simulink model "Tmod_PID_ObsMej_Simulacion"  (R2021a)
settings: Solver=VariableStepAuto  StartTime=0.0  StopTime=20  MaxStep=1e-4  RelTol=1e-3
values from neighbouring files (symbols this model uses):
  a1c = -A1(2, 2)    [filtros_ss.m]
  a1m = -A4(2, 2)    [filtros_ss.m]
  a1p = -A2(2, 2)    [filtros_ss.m]
  a1t = -A3    [filtros_ss.m]
  a2c = -A1(2, 1)    [filtros_ss.m]
  a2m = -A4(2, 1)    [filtros_ss.m]
  a2p = -A2(2, 1)    [filtros_ss.m]
  a_cu = 3.9e-3    (= 0.0039)    [Datos.m]
  b_eq = 15.000e-6    (= 1.5e-05)    [Datos.m]
  ba = 0.0113    [Datos.m]
  Cts = 0.818    [Datos.m]
  Id_0 = 0    [Datos.m]
  J_eq = 5.6509e-6    (= 5.6509e-06)    [Datos.m]
  Ksa = 9.0414    [Datos.m]
  Ksia = 2893.2608    [Datos.m]
  lambda_m = 0.01546    [Datos.m]
  Ld = 6.6e-3    (= 0.0066)    [Datos.m]
  Lls = 0.8e-3    (= 0.0008)    [Datos.m]
  Lq = 5.8e-3    (= 0.0058)    [Datos.m]
  Pp = 3.01    [Datos.m]
  r = 314.3008    [Datos.m]
  Rs = 1.02    [Datos.m]
  Rs_ref = 1.02    [Datos.m]
  Rtsamb = 146.7    [Datos.m]
  sat = sqrt(2/3)*24    [filtros_ss.m]
  T_0 = 40.0    (= 40)    [Datos.m]
  T_amb = 40    [Datos.m]
  Tlmax = 6.28    [Datos.m]
  Ts_ref = 40    [Datos.m]
undefined symbols (not defined in the file or in its folder): A1, A2, A3, B1, B2, B3, C1, C2, C3, D1, D2, D3, mKi, mKtheta, mKw, R0, Rd, Rq, sigbuilder_block
libraries: simulink x1
settings Model: Creator=ThnkPad  LastModifiedBy=jpss8

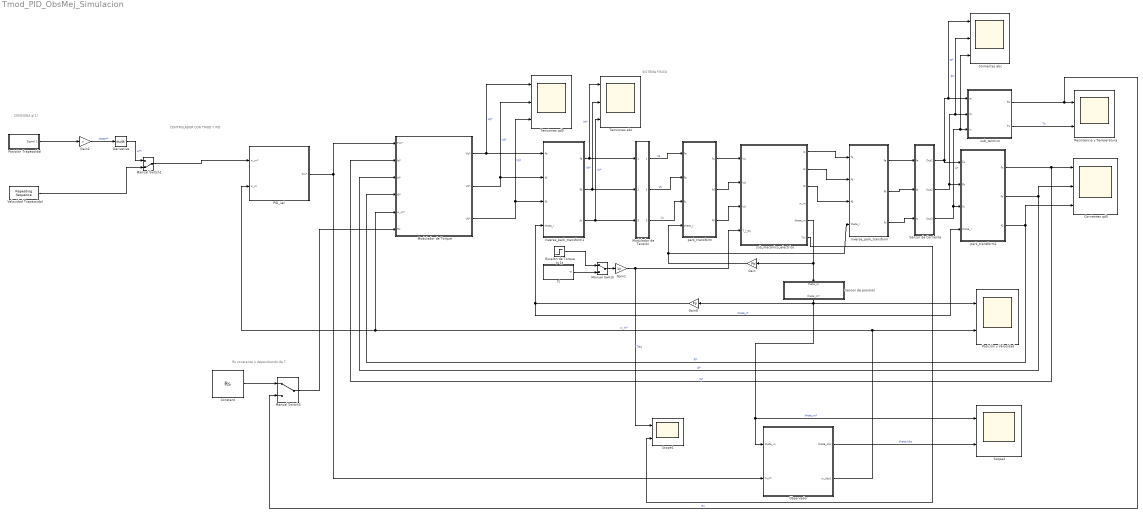
== system Tmod_PID_ObsMej_Simulacion ==
  note: Rs constante o dependiendo de T
  note: CONSIGNA q(1)
  note: CONTROLADOR CON TMOD Y PID
  note: SISTEMA FÍSICO
  Constant : Constant  Value=Rs
  Corrientes abc : Scope  NumInputPorts=3
  Corrientes qd0 : Scope  NumInputPorts=3
  Derivative : Derivative
  Escalón de Torque t=1s : Step  After=Tlmax  SampleTime=0
  Gain : Gain  Gain=Pp
  Gain1 : Gain  Gain=1/r
  Gain2 : Gain  Gain=r
  Gain8 : Gain  Gain=Pp
  Manual Switch : ManualSwitch
  Manual Switch1 : ManualSwitch  CurrentSetting=0
  Manual Switch3 : ManualSwitch
  Modulador de Tensión : Subsystem
  Modulador de Torque : Subsystem
  Observador : Subsystem
  PID_vel : Subsystem
  Posición Trapezoidal : Subsystem  Tag=STV Subsys  LoadFcn=sigbuilder_block('load');  StartFcn=sigbuilder_block('start');  StopFcn=sigbuilder_block('stop');  ClipboardFcn=sigbuilder_block('clipboard');  mask(Sigbuilder block){tuvar=[0:10]}
      mask help: Simulink:masks:SigbuilderBlock_MD
      mask init:
      | if ~strcmp(get_param(bdroot(gcbh),'SimulationStatus'),'stopped') tuvar = sigbuilder_block('maskInit'); end
      settings: CopyFcn=sigbuilder_block('copy');  DeleteFcn=sigbuilder_block('delete');  ModelCloseFcn=sigbuilder_block('modelClose');  PreSaveFcn=sigbuilder_block('preSave');  PauseFcn=sigbuilder_block('pause');  ContinueFcn=sigbuilder_block('continue');  NameChangeFcn=sigbuilder_block('namechange');  OpenFcn=sigbuilder_block('open',[-53.25 9 1012.5 477.75 ]);  CloseFcn=sigbuilder_block('close');
      mask Display: plot(0, 0, 100, 100,[2, 2, 32, 32, 2], [68, 8, 8, 68, 68],[32, 2], [38, 38], [32, 19, 2],[53, 60, 44], [32, 17, 17, 2],[16, 16, 31, 31]);txt = getActiveGroup(gcbh);text(2, 100, txt,'verticalAlignment', 'top');
  Posición y Velocidad : Scope  NumInputPorts=2
  Resistencia y Temperatura : Scope  NumInputPorts=2
  Scope1 : Scope  NumInputPorts=2
  Scope2 : Scope  NumInputPorts=2
  Sensor de Corriente : Subsystem
  Sensor de posicion : Subsystem
      settings: PortSchema="{\"entries\":[{\"content\":{\"sides\":[{\"content\":{\"connectorIds\":[]},\"type\":\"ConnectorPlacement.EquallySpacedRectSide\",\"uuid\":\"b536d0fd-a8b9-4fb9-bd2d-8cdbea63ffed\"},{\"content\":{\"connectorIds\":[],\"side\":\"RIGHT\"},\"type\":\"ConnectorPlacement.EquallySpacedRectSide\",\"uuid\":\"53663a0b-a681-499d-8c35-4379374d5e5a\"},{\"content\":{\"connectorIds\":[\"In1\"],\"side\":\"TOP\"},\"type\":\"ConnectorPlacement.EquallySpacedRectSide\",\"uuid\":\"1d4df5dd-d4dd-4e51-a644-5027fa847818\"},{\"content\":{\"connectorIds\":[\"Out1\"],\"side\":\"BOTTOM\"},\"type\":\"ConnectorPlacement.EquallySpacedRectSide\",\"uuid\":\"bae52777-b033-4852-a05b-da4dd91f0167\"}]},\"type\":\"ConnectorPlacement.EquallySpacedConnector\",\"uuid\":\"afdb905b-2ae6-4e5d-8f00-48d2cd8bae21\"}],\"packageUris\":[\"http://schema.mathworks.com/mf0/Connector/R2020b\"],\"version\":\"1.0\"}"
  Tensiones abc : Scope  NumInputPorts=3
  Tensiones qd0 : Scope  NumInputPorts=3
  Tl : Subsystem  Tag=STV Subsys  LoadFcn=sigbuilder_block('load');  StartFcn=sigbuilder_block('start');  StopFcn=sigbuilder_block('stop');  ClipboardFcn=sigbuilder_block('clipboard');  mask(Sigbuilder block){tuvar=[0:10]}
      mask help: Simulink:masks:SigbuilderBlock_MD
      mask init:
      | if ~strcmp(get_param(bdroot(gcbh),'SimulationStatus'),'stopped') tuvar = sigbuilder_block('maskInit'); end
      settings: CopyFcn=sigbuilder_block('copy');  DeleteFcn=sigbuilder_block('delete');  ModelCloseFcn=sigbuilder_block('modelClose');  PreSaveFcn=sigbuilder_block('preSave');  PauseFcn=sigbuilder_block('pause');  ContinueFcn=sigbuilder_block('continue');  NameChangeFcn=sigbuilder_block('namechange');  OpenFcn=sigbuilder_block('open',[6 0 1012.5 477.75 ]);  CloseFcn=sigbuilder_block('close');
      mask Display: plot(0, 0, 100, 100,[2, 2, 32, 32, 2], [68, 8, 8, 68, 68],[32, 2], [38, 38], [32, 19, 2],[53, 60, 44], [32, 17, 17, 2],[16, 16, 31, 31]);txt = getActiveGroup(gcbh);text(2, 100, txt,'verticalAlignment', 'top');
  Velocidad Trapezoidal : simulink/Sources/Repeating Sequence  rep_seq_t=t_sequence  rep_seq_y=w2
  inverse_park_transform : MATLAB Function  TreatAsAtomicUnit=on
  inverse_park_transform1 : MATLAB Function  TreatAsAtomicUnit=on
  park_transform : MATLAB Function  TreatAsAtomicUnit=on
  park_transform1 : MATLAB Function  TreatAsAtomicUnit=on
  sub_mecanico_electrico : Subsystem
  sub_termico : Subsystem
  wires:
  Sensor de Corriente/3(Out3) -> park_transform1/3(fc), Corrientes abc/3, sub_termico/3(ic)  "Ic*"
  sub_termico/2(Ts) -> Resistencia y Temperatura/2  "Ts"
  inverse_park_transform1/2(fb) -> Modulador de Tensión/2(Vb), Tensiones abc/2  "Vb*"
  Modulador de Torque/2(Vd*) -> Tensiones qd0/2, inverse_park_transform1/2(fd)  "Vd*"
  Sensor de Corriente/2(Out2) -> park_transform1/2(fb), Corrientes abc/2, sub_termico/2(ib)  "Ib*"
  PID_vel/1(Tm*) -> Modulador de Torque/1(Tm*'), Observador/2(Tm**)
  park_transform1/3(f0) -> Corrientes qd0/3, Modulador de Torque/4(I0*)  "I0*"
  park_transform1/1(fq) -> Modulador de Torque/2(Iq*), Corrientes qd0/1  "Iq*"
  inverse_park_transform1/1(fa) -> Tensiones abc/1, Modulador de Tensión/1(Va)  "Va*"
  Modulador de Torque/3(V0*) -> inverse_park_transform1/3(f0), Tensiones qd0/3  "V0*"
  Gain/1 -> inverse_park_transform/4(theta_r), park_transform/4(theta_r)
  sub_mecanico_electrico/5(theta_m) -> Sensor de posicion/1(theta_m), Gain/1
  inverse_park_transform1/3(fc) -> Modulador de Tensión/3(Vc), Tensiones abc/3  "Vc*"
  inverse_park_transform/1(fa) -> Sensor de Corriente/1(Ia)
  inverse_park_transform/3(fc) -> Sensor de Corriente/3(Ic)
  park_transform/2(fd) -> sub_mecanico_electrico/2(Vd)
  sub_mecanico_electrico/1(iq) -> inverse_park_transform/1(fq)
  park_transform1/2(fd) -> Corrientes qd0/2, Modulador de Torque/3(Id*)  "Id*"
  Gain8/1 -> park_transform1/4(theta_r), inverse_park_transform1/4(theta_r)  "theta_r*"
  park_transform/1(fq) -> sub_mecanico_electrico/1(Vq)
  park_transform/3(f0) -> sub_mecanico_electrico/3(V0)
  Sensor de posicion/1(theta_m*) -> Posición y Velocidad/1, Scope2/1, Observador/1(theta_m), Gain8/1  "theta_m*"
  Modulador de Torque/1(Vq*) -> Tensiones qd0/1, inverse_park_transform1/1(fq)  "Vq*"
  Modulador de Tensión/3(Vc*) -> park_transform/3(fc)  "Vc"
  Sensor de Corriente/1(Out1) -> park_transform1/1(fa), Corrientes abc/1, sub_termico/1(ia)  "Ia*"
  inverse_park_transform/2(fb) -> Sensor de Corriente/2(Ib)
  sub_termico/1(Rs) -> Resistencia y Temperatura/1, Manual Switch3/2  "Rs"
  Modulador de Tensión/1(Va*) -> park_transform/1(fa)  "Va"
  Observador/2(w_obs1) -> PID_vel/2(w_m), Modulador de Torque/5(w_m*), Posición y Velocidad/2  "w_m*"
  Modulador de Tensión/2(Vb*) -> park_transform/2(fb)  "Vb"
  sub_mecanico_electrico/3(i0) -> inverse_park_transform/3(f0)
  Gain1/1 -> Scope1/1, sub_mecanico_electrico/4(T_l_eq)  "Tleq"
  sub_mecanico_electrico/2(id) -> inverse_park_transform/2(fd)
  Gain2/1 -> Derivative/1  "theta**"
  sub_mecanico_electrico/6(Tm) -> Scope1/2
  Observador/1(theta_obs) -> Scope2/2  "theta_obs"
  Tl/1(Tl) -> Manual Switch/2
  Escalón de Torque t=1s/1 -> Manual Switch/1
  Posición Trapezoidal/1(Signal 1) -> Gain2/1
  Constant/1 -> Manual Switch3/1
  Manual Switch3/1 -> Modulador de Torque/6(Rs)
  Manual Switch1/1 -> PID_vel/1(w_m*)
  Derivative/1 -> Manual Switch1/1  "w**"
  Velocidad Trapezoidal/1 -> Manual Switch1/2
  Manual Switch/1 -> Gain1/1

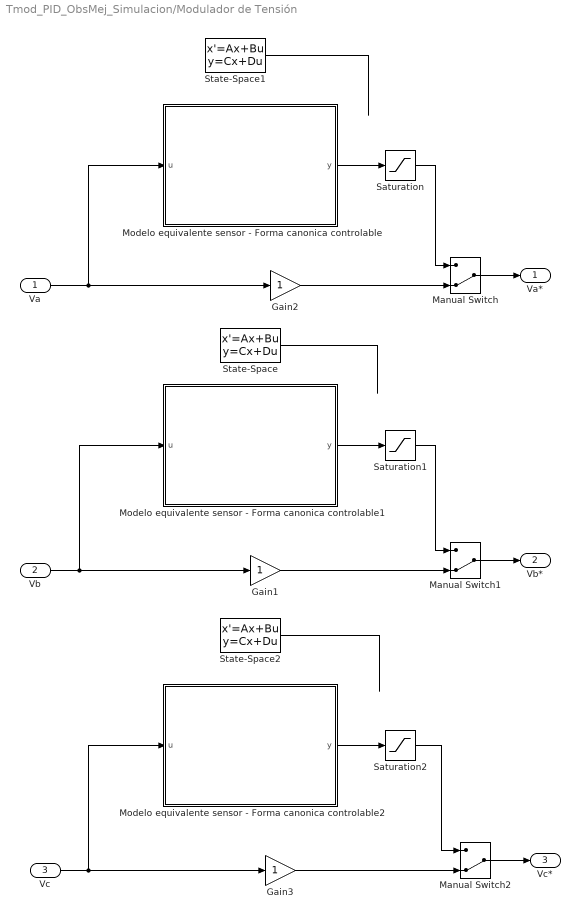
== system Tmod_PID_ObsMej_Simulacion/Modulador de Tensión ==
  Va : Inport
  Vb : Inport  Port=2
  Vc : Inport  Port=3
  Gain1 : Gain
  Gain2 : Gain
  Gain3 : Gain
  Manual Switch : ManualSwitch  CurrentSetting=0
  Manual Switch1 : ManualSwitch  CurrentSetting=0
  Manual Switch2 : ManualSwitch  CurrentSetting=0
  Modelo equivalente sensor - Forma canonica controlable : Subsystem
  Modelo equivalente sensor - Forma canonica controlable1 : Subsystem
  Modelo equivalente sensor - Forma canonica controlable2 : Subsystem
  Saturation : Saturate  UpperLimit=sat  LowerLimit=-sat
  Saturation1 : Saturate  UpperLimit=sat  LowerLimit=-sat
  Saturation2 : Saturate  UpperLimit=sat  LowerLimit=-sat
  State-Space : StateSpace  A=A1  B=B1  C=C1  D=D1  InitialCondition=0
  State-Space1 : StateSpace  A=A1  B=B1  C=C1  D=D1  InitialCondition=0
  State-Space2 : StateSpace  A=A1  B=B1  C=C1  D=D1  InitialCondition=0
  Va* : Outport
  Vb* : Outport  Port=2
  Vc* : Outport  Port=3
  wires:
  Va/1 -> Modelo equivalente sensor - Forma canonica controlable/1(u), Gain2/1
  Manual Switch/1 -> Va*/1
  Gain2/1 -> Manual Switch/2
  Vb/1 -> Modelo equivalente sensor - Forma canonica controlable1/1(u), Gain1/1
  Manual Switch1/1 -> Vb*/1
  Gain1/1 -> Manual Switch1/2
  Vc/1 -> Modelo equivalente sensor - Forma canonica controlable2/1(u), Gain3/1
  Manual Switch2/1 -> Vc*/1
  Gain3/1 -> Manual Switch2/2
  Saturation/1 -> Manual Switch/1
  Saturation1/1 -> Manual Switch1/1
  Saturation2/1 -> Manual Switch2/1
  State-Space/1 -> ?
  State-Space1/1 -> ?
  State-Space2/1 -> ?
  Modelo equivalente sensor - Forma canonica controlable/1(y) -> Saturation/1
  Modelo equivalente sensor - Forma canonica controlable1/1(y) -> Saturation1/1
  Modelo equivalente sensor - Forma canonica controlable2/1(y) -> Saturation2/1

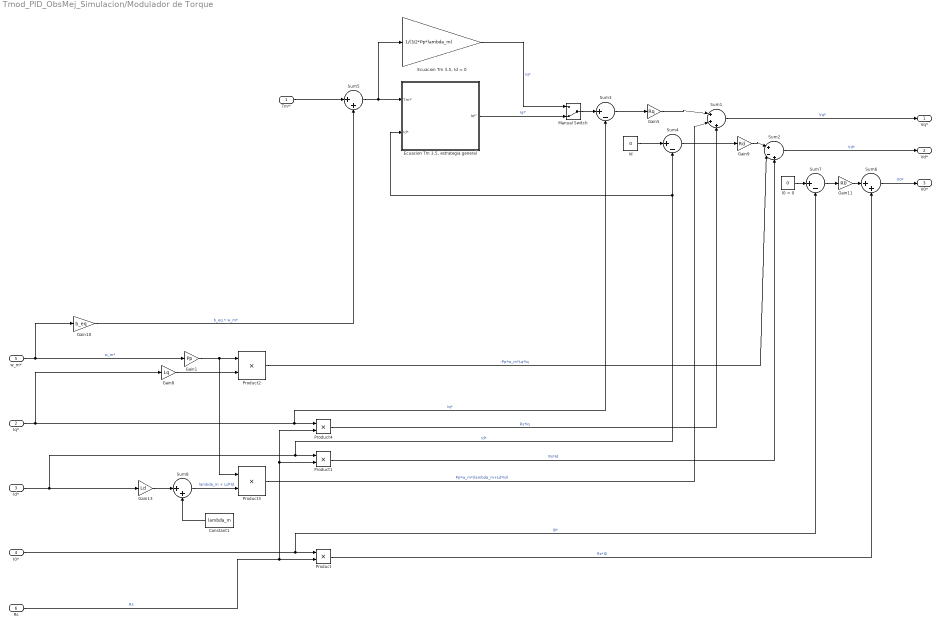
== system Tmod_PID_ObsMej_Simulacion/Modulador de Torque ==
  Tm*' : Inport
  Iq* : Inport  Port=2
  Id* : Inport  Port=3
  I0* : Inport  Port=4
  w_m* : Inport  Port=5
  Rs : Inport  Port=6
  Constant1 : Constant  Value=lambda_m
  "Ecuacion Tm 3.5, Id = 0" : Gain  Gain=1/(3/2*Pp*lambda_m)
  "Ecuacion Tm 3.5, estrategia general" : Subsystem
  Gain1 : Gain  Gain=Pp
  Gain10 : Gain  Gain=b_eq
  Gain11 : Gain  Gain=R0
  Gain13 : Gain  Gain=Ld
  Gain5 : Gain  Gain=Rq
  Gain8 : Gain  Gain=Lq
  Gain9 : Gain  Gain=Rd
  I0 = 0 : Constant  Value=0
  Id : Constant  Value=0
  Manual Switch : ManualSwitch  CurrentSetting=0
  Product{,1..4} (5 alike) : Product
  Sum1 : Sum  Inputs=|+++
  Sum2 : Sum  Inputs=|+-+
  Sum3 : Sum  Inputs=|+-
  Sum4 : Sum  Inputs=|+-
  Sum5 : Sum  Inputs=|++
  Sum6 : Sum  Inputs=|++
  Sum7 : Sum  Inputs=|+-
  Sum8 : Sum  Inputs=|++
  Vq* : Outport
  Vd* : Outport  Port=2
  V0* : Outport  Port=3
  wires:
  Sum7/1 -> Gain11/1
  I0 = 0/1 -> Sum7/1
  Tm*'/1 -> Sum5/1
  "Ecuacion Tm 3.5, Id = 0"/1 -> Manual Switch/1  "Iq*"
  Sum4/1 -> Gain9/1
  Sum5/1 -> "Ecuacion Tm 3.5, Id = 0"/1, "Ecuacion Tm 3.5, estrategia general"/1(Tm*')
  Id/1 -> Sum4/1
  Gain5/1 -> Sum1/1
  Gain9/1 -> Sum2/1
  Sum3/1 -> Gain5/1
  Sum2/1 -> Vd*/1  "Vd*"
  Gain11/1 -> Sum6/1
  Sum1/1 -> Vq*/1  "Vq*"
  Gain10/1 -> Sum5/2  "b_eq * w_m*"
  Product4/1 -> Sum1/3  "Rs*Iq"
  Product2/1 -> Sum2/2  "-Pp*w_m*Lq*Iq"
  Product1/1 -> Sum2/3  "Rs*Id"
  Product/1 -> Sum6/2  "Rs*I0"
  Product3/1 -> Sum1/2  "Pp*w_m*(lambda_m+Ld*Id)"
  w_m*/1 -> Gain10/1, Gain1/1  "w_m*"
  Iq*/1 -> Product4/1, Sum3/2, Gain8/1  "Iq*"
  Gain13/1 -> Sum8/1
  Gain8/1 -> Product2/2
  Gain1/1 -> Product3/1, Product2/1
  Constant1/1 -> Sum8/2
  Sum8/1 -> Product3/2  "lambda_m + Ld*Id"
  Id*/1 -> Product1/1, "Ecuacion Tm 3.5, estrategia general"/2(Id*), Sum4/2, Gain13/1  "Id*"
  I0*/1 -> Product/1, Sum7/2  "I0*"
  Sum6/1 -> V0*/1  "V0*"
  "Ecuacion Tm 3.5, estrategia general"/1(Iq*') -> Manual Switch/2  "Iq*'"
  Manual Switch/1 -> Sum3/1
  Rs/1 -> Product1/2, Product4/2, Product/2  "Rs"

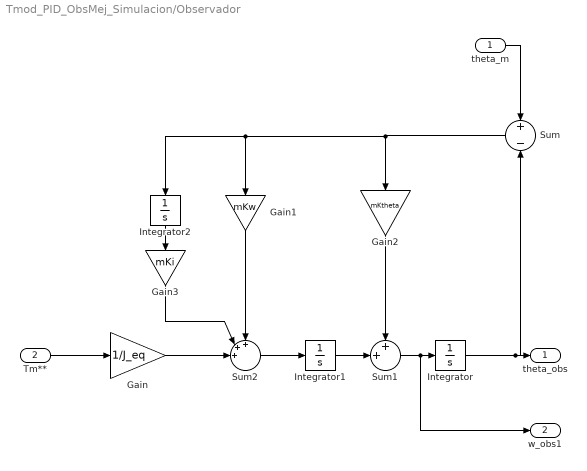
== system Tmod_PID_ObsMej_Simulacion/Observador ==
  theta_m : Inport
  Tm** : Inport  Port=2
  Gain : Gain  Gain=1/J_eq
  Gain1 : Gain  Gain=mKw
  Gain2 : Gain  Gain=mKtheta
  Gain3 : Gain  Gain=mKi
  Integrator : Integrator
  Integrator1 : Integrator
  Integrator2 : Integrator
  Sum : Sum  Inputs=+|-
  Sum1 : Sum  Inputs=++|
  Sum2 : Sum  Inputs=+++||
  theta_obs : Outport
  w_obs1 : Outport  Port=2
  wires:
  Integrator/1 -> Sum/2, theta_obs/1
  Sum2/1 -> Integrator1/1
  Sum/1 -> Integrator2/1, Gain1/1, Gain2/1
  theta_m/1 -> Sum/1
  Tm**/1 -> Gain/1
  Gain1/1 -> Sum2/1
  Gain2/1 -> Sum1/1
  Integrator1/1 -> Sum1/2
  Sum1/1 -> w_obs1/1, Integrator/1
  Gain/1 -> Sum2/3
  Gain3/1 -> Sum2/2
  Integrator2/1 -> Gain3/1

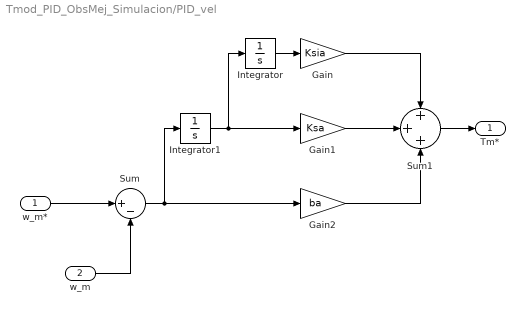
== system Tmod_PID_ObsMej_Simulacion/PID_vel ==
  w_m* : Inport
  w_m : Inport  Port=2
  Gain : Gain  Gain=Ksia
  Gain1 : Gain  Gain=Ksa
  Gain2 : Gain  Gain=ba
  Integrator : Integrator
  Integrator1 : Integrator
  Sum : Sum  Inputs=|+-
  Sum1 : Sum  Inputs=+++
  Tm* : Outport
  wires:
  Gain1/1 -> Sum1/2
  Sum1/1 -> Tm*/1
  Sum/1 -> Integrator1/1, Gain2/1
  Integrator/1 -> Gain/1
  Gain2/1 -> Sum1/3
  Gain/1 -> Sum1/1
  Integrator1/1 -> Gain1/1, Integrator/1
  w_m*/1 -> Sum/1
  w_m/1 -> Sum/2

== system Tmod_PID_ObsMej_Simulacion/Posición Trapezoidal ==
  Demux : Demux  Tag=STV Demux  Outputs=1
      settings: DisplayOption=none
  FromWs : FromWorkspace  Tag=STV FromWs  VariableName=tuvar
      SigBuilderData=|
      | common.afterFinalStr = 'Extrapolate'
      | common.sampleTime = 0
      | dataSet.timeRange = [0 20]
      | dataSet.name = 'Group 1'
      | sbobj.Groups.Name = 'Group 1'
      | sbobj.Groups.Signals.Name = 'Signal 1'
      | sbobj.Groups.Signals.XData = [0 2 7 12 17 20]
      | sbobj.Groups.Signals.YData = [0 0 6.28318530718 6.28318530718 0 0]
      | sbobj.Groups.TimeRange = [0 20]
  Signal 1 : Outport  Tag=STV Outport
  wires:
  Demux/1 -> Signal 1/1
  FromWs/1 -> Demux/1

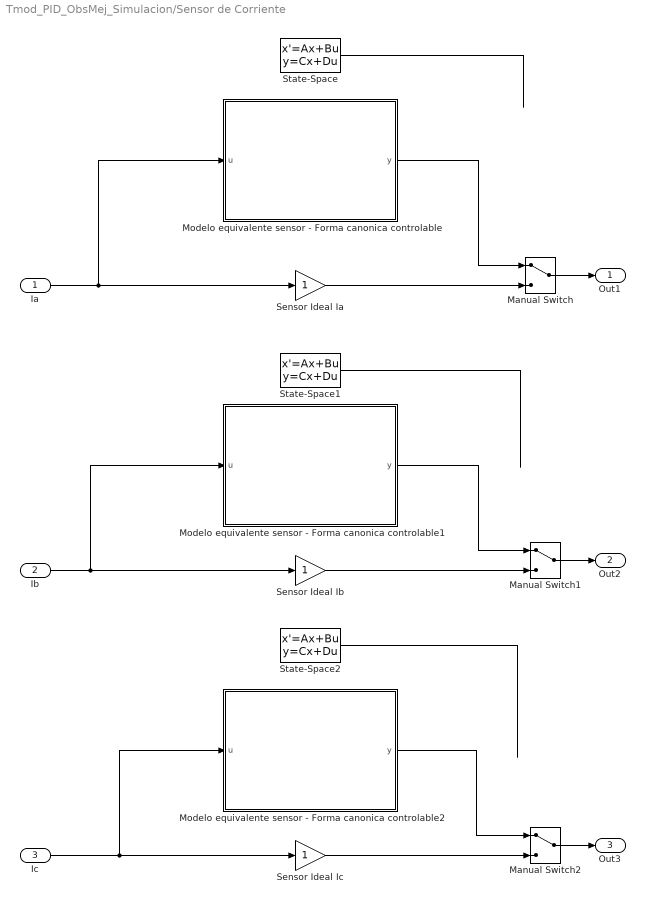
== system Tmod_PID_ObsMej_Simulacion/Sensor de Corriente ==
  Ia : Inport
  Ib : Inport  Port=2
  Ic : Inport  Port=3
  Manual Switch : ManualSwitch
  Manual Switch1 : ManualSwitch
  Manual Switch2 : ManualSwitch
  Modelo equivalente sensor - Forma canonica controlable : Subsystem
  Modelo equivalente sensor - Forma canonica controlable1 : Subsystem
  Modelo equivalente sensor - Forma canonica controlable2 : Subsystem
  Sensor Ideal Ia : Gain
  Sensor Ideal Ib : Gain
  Sensor Ideal Ic : Gain
  State-Space : StateSpace  A=A1  B=B1  C=C1  D=D1  InitialCondition=0
  State-Space1 : StateSpace  A=A1  B=B1  C=C1  D=D1  InitialCondition=0
  State-Space2 : StateSpace  A=A1  B=B1  C=C1  D=D1  InitialCondition=0
  Out1 : Outport
  Out2 : Outport  Port=2
  Out3 : Outport  Port=3
  wires:
  Ic/1 -> Modelo equivalente sensor - Forma canonica controlable2/1(u), Sensor Ideal Ic/1
  Ib/1 -> Modelo equivalente sensor - Forma canonica controlable1/1(u), Sensor Ideal Ib/1
  Ia/1 -> Modelo equivalente sensor - Forma canonica controlable/1(u), Sensor Ideal Ia/1
  Manual Switch/1 -> Out1/1
  Sensor Ideal Ia/1 -> Manual Switch/2
  Manual Switch2/1 -> Out3/1
  Manual Switch1/1 -> Out2/1
  Sensor Ideal Ib/1 -> Manual Switch1/2
  Sensor Ideal Ic/1 -> Manual Switch2/2
  State-Space/1 -> ?
  State-Space1/1 -> ?
  State-Space2/1 -> ?
  Modelo equivalente sensor - Forma canonica controlable/1(y) -> Manual Switch/1
  Modelo equivalente sensor - Forma canonica controlable1/1(y) -> Manual Switch1/1
  Modelo equivalente sensor - Forma canonica controlable2/1(y) -> Manual Switch2/1

== system Tmod_PID_ObsMej_Simulacion/Sensor de posicion ==
  theta_m : Inport
  Manual Switch : ManualSwitch
  Modelo equivalente sensor - Forma canonica controlable : Subsystem
  Sensor Ideal : Gain
  State-Space : StateSpace  A=A2  B=B2  C=C2  D=D2  InitialCondition=0
  theta_m* : Outport
  wires:
  theta_m/1 -> Modelo equivalente sensor - Forma canonica controlable/1(u), Sensor Ideal/1
  Manual Switch/1 -> theta_m*/1
  Sensor Ideal/1 -> Manual Switch/2
  Modelo equivalente sensor - Forma canonica controlable/1(y) -> Manual Switch/1
  State-Space/1 -> ?

== system Tmod_PID_ObsMej_Simulacion/Tl ==
  Demux : Demux  Tag=STV Demux  Outputs=1
      settings: DisplayOption=none
  FromWs : FromWorkspace  Tag=STV FromWs  VariableName=tuvar
      SigBuilderData=|
      | common.afterFinalStr = 'Extrapolate'
      | common.sampleTime = 0
      | dataSet.timeRange = [0 1]
      | dataSet.name = 'Group 1'
      | sbobj.Groups.Name = 'Group 1'
      | sbobj.Groups.Signals.Name = 'Tl'
      | sbobj.Groups.Signals.XData = [0 0.3 0.3 0.5 0.5 0.9 0.9 1]
      | sbobj.Groups.Signals.YData = [0 0 6.28 6.28 -6.28 -6.28 0 0]
      | sbobj.Groups.TimeRange = [0 1]
  Tl : Outport  Tag=STV Outport
  wires:
  FromWs/1 -> Demux/1
  Demux/1 -> Tl/1

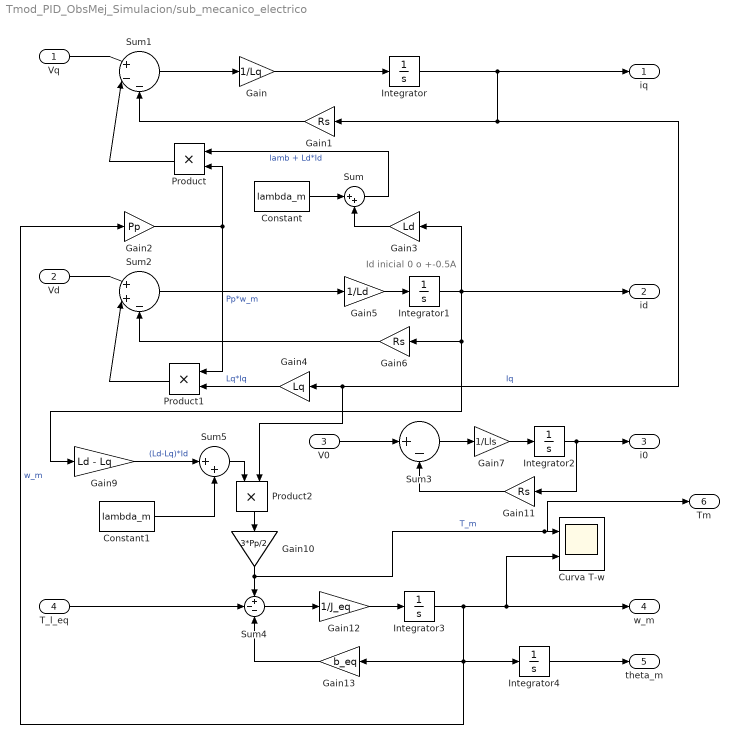
== system Tmod_PID_ObsMej_Simulacion/sub_mecanico_electrico ==
  note: Id inicial 0 o +-0.5A
  Vq : Inport
  Vd : Inport  Port=2
  V0 : Inport  Port=3
  T_l_eq : Inport  Port=4
  Constant : Constant  Value=lambda_m
  Constant1 : Constant  Value=lambda_m
  Curva T-w : Scope  NumInputPorts=2
  Gain : Gain  Gain=1/Lq
  Gain1 : Gain  Gain=Rs
  Gain10 : Gain  Gain=3*Pp/2
  Gain11 : Gain  Gain=Rs
  Gain12 : Gain  Gain=1/J_eq
  Gain13 : Gain  Gain=b_eq
  Gain2 : Gain  Gain=Pp
  Gain3 : Gain  Gain=Ld
  Gain4 : Gain  Gain=Lq
  Gain5 : Gain  Gain=1/Ld
  Gain6 : Gain  Gain=Rs
  Gain7 : Gain  Gain=1/Lls
  Gain9 : Gain  Gain=Ld - Lq
  Integrator{,2..4} (4 alike) : Integrator
  Integrator1 : Integrator  InitialCondition=Id_0
  Product : Product
  Product1 : Product
  Product2 : Product
  Sum : Sum  Inputs=|++
  Sum1 : Sum  Inputs=|+--
  Sum2 : Sum  Inputs=|++-
  Sum3 : Sum  Inputs=|+-
  Sum4 : Sum  Inputs=+--
  Sum5 : Sum  Inputs=|++
  iq : Outport
  id : Outport  Port=2
  i0 : Outport  Port=3
  w_m : Outport  Port=4
  theta_m : Outport  Port=5
  Tm : Outport  Port=6
  wires:
  Gain12/1 -> Integrator3/1
  T_l_eq/1 -> Sum4/2
  Sum4/1 -> Gain12/1
  Gain10/1 -> Tm/1, Curva T-w/1, Sum4/1  "T_m"
  Integrator4/1 -> theta_m/1
  Gain13/1 -> Sum4/3
  Integrator3/1 -> Gain2/1, Integrator4/1, Gain13/1, Curva T-w/2, w_m/1  "w_m"
  Constant1/1 -> Sum5/2
  Gain9/1 -> Sum5/1  "(Ld-Lq)*Id"
  Sum5/1 -> Product2/1
  Product2/1 -> Gain10/1
  V0/1 -> Sum3/1
  Gain11/1 -> Sum3/2
  Gain5/1 -> Integrator1/1
  Sum2/1 -> Gain5/1
  Integrator1/1 -> Gain9/1, Gain6/1, id/1, Gain3/1
  Product/1 -> Sum1/2
  Integrator2/1 -> i0/1, Gain11/1
  Product1/1 -> Sum2/2
  Gain4/1 -> Product1/2  "Lq*Iq"
  Gain1/1 -> Sum1/3
  Gain6/1 -> Sum2/3
  Sum/1 -> Product/1  "lamb + Ld*Id"
  Sum3/1 -> Gain7/1
  Gain7/1 -> Integrator2/1
  Vd/1 -> Sum2/1
  Gain3/1 -> Sum/2
  Gain2/1 -> Product1/1, Product/2  "Pp*w_m"
  Integrator/1 -> Gain1/1, Gain4/1, Product2/2, iq/1  "Iq"
  Sum1/1 -> Gain/1
  Gain/1 -> Integrator/1
  Constant/1 -> Sum/1
  Vq/1 -> Sum1/1

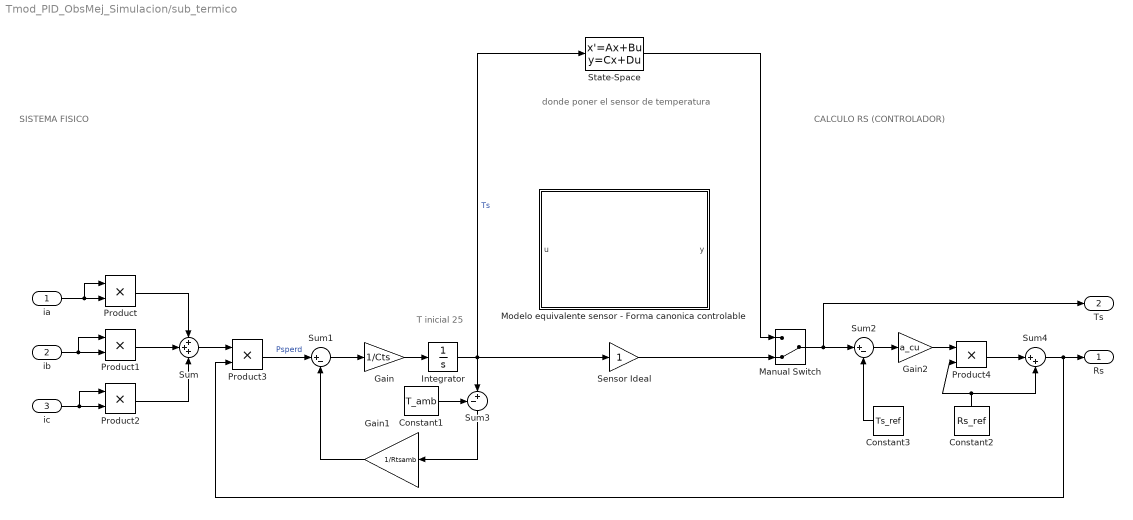
== system Tmod_PID_ObsMej_Simulacion/sub_termico ==
  note: CALCULO RS (CONTROLADOR)
  note: SISTEMA FISICO
  note: donde poner el sensor de temperatura
  note: T inicial 25
  ia : Inport
  ib : Inport  Port=2
  ic : Inport  Port=3
  Constant1 : Constant  Value=T_amb
  Constant2 : Constant  Value=Rs_ref
  Constant3 : Constant  Value=Ts_ref
  Gain : Gain  Gain=1/Cts
  Gain1 : Gain  Gain=1/Rtsamb
  Gain2 : Gain  Gain=a_cu
  Integrator : Integrator  InitialCondition=T_0
  Manual Switch : ManualSwitch  CurrentSetting=0
  Modelo equivalente sensor - Forma canonica controlable : Subsystem
  Product{,1..4} (5 alike) : Product
  Sensor Ideal : Gain
  State-Space : StateSpace  A=A3  B=B3  C=C3  D=D3  InitialCondition=T_0
  Sum : Sum  Inputs=+++
  Sum1 : Sum  Inputs=|+-
  Sum2 : Sum  Inputs=|+-
  Sum3 : Sum  Inputs=-+|
  Sum4 : Sum  Inputs=|++
  Rs : Outport
  Ts : Outport  Port=2
  wires:
  ic/1 -> Product2/1, Product2/2
  ib/1 -> Product1/1, Product1/2
  ia/1 -> Product/1, Product/2
  Product/1 -> Sum/1
  Product1/1 -> Sum/2
  Product2/1 -> Sum/3
  Product3/1 -> Sum1/1  "Psperd"
  Sum/1 -> Product3/1
  Sum4/1 -> Product3/2, Rs/1
  Gain1/1 -> Sum1/2
  Gain/1 -> Integrator/1
  Sum1/1 -> Gain/1
  Integrator/1 -> State-Space/1, Sensor Ideal/1, Sum3/2  "Ts"
  Sum3/1 -> Gain1/1
  Constant1/1 -> Sum3/1
  Sum2/1 -> Gain2/1
  Gain2/1 -> Product4/1
  Product4/1 -> Sum4/1
  Constant2/1 -> Product4/2, Sum4/2
  Constant3/1 -> Sum2/2
  Manual Switch/1 -> Ts/1, Sum2/1
  Sensor Ideal/1 -> Manual Switch/2
  State-Space/1 -> Manual Switch/1

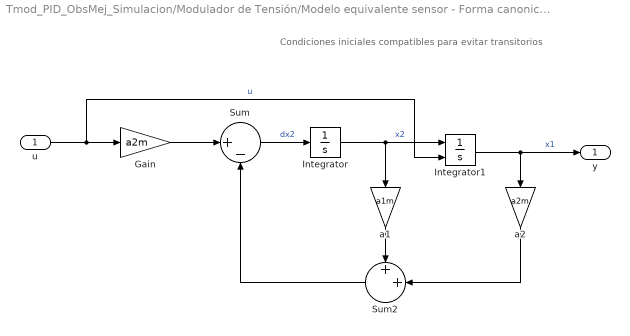
== system Tmod_PID_ObsMej_Simulacion/Modulador de Tensión/Modelo equivalente sensor - Forma canonica controlable ==
  note: Condiciones iniciales compatibles para evitar transitorios
  u : Inport
  Gain : Gain  Gain=a2m
  Integrator : Integrator
  Integrator1 : Integrator  InitialConditionSource=external
  Sum : Sum  Inputs=|+-
  Sum2 : Sum  Inputs=++|
  a1 : Gain  Gain=a1m
  a2 : Gain  Gain=a2m
  y : Outport
  wires:
  Sum/1 -> Integrator/1  "dx2"
  Integrator/1 -> a1/1, Integrator1/1  "x2"
  a1/1 -> Sum2/1
  Integrator1/1 -> y/1, a2/1  "x1"
  a2/1 -> Sum2/2
  Sum2/1 -> Sum/2
  u/1 -> Integrator1/2, Gain/1  "u"
  Gain/1 -> Sum/1

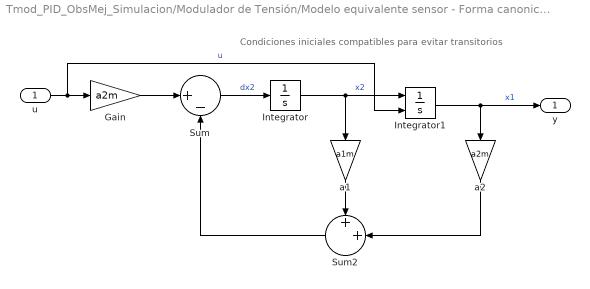
== system Tmod_PID_ObsMej_Simulacion/Modulador de Tensión/Modelo equivalente sensor - Forma canonica controlable1 ==
  note: Condiciones iniciales compatibles para evitar transitorios
  u : Inport
  Gain : Gain  Gain=a2m
  Integrator : Integrator
  Integrator1 : Integrator  InitialConditionSource=external
  Sum : Sum  Inputs=|+-
  Sum2 : Sum  Inputs=++|
  a1 : Gain  Gain=a1m
  a2 : Gain  Gain=a2m
  y : Outport
  wires:
  Sum/1 -> Integrator/1  "dx2"
  Integrator/1 -> a1/1, Integrator1/1  "x2"
  a1/1 -> Sum2/1
  Integrator1/1 -> y/1, a2/1  "x1"
  a2/1 -> Sum2/2
  Sum2/1 -> Sum/2
  u/1 -> Integrator1/2, Gain/1  "u"
  Gain/1 -> Sum/1

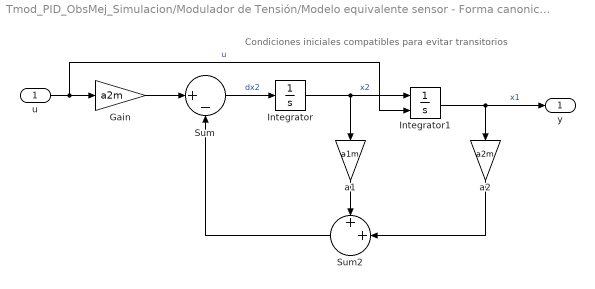
== system Tmod_PID_ObsMej_Simulacion/Modulador de Tensión/Modelo equivalente sensor - Forma canonica controlable2 ==
  note: Condiciones iniciales compatibles para evitar transitorios
  u : Inport
  Gain : Gain  Gain=a2m
  Integrator : Integrator
  Integrator1 : Integrator  InitialConditionSource=external
  Sum : Sum  Inputs=|+-
  Sum2 : Sum  Inputs=++|
  a1 : Gain  Gain=a1m
  a2 : Gain  Gain=a2m
  y : Outport
  wires:
  Sum/1 -> Integrator/1  "dx2"
  Integrator/1 -> a1/1, Integrator1/1  "x2"
  a1/1 -> Sum2/1
  Integrator1/1 -> y/1, a2/1  "x1"
  a2/1 -> Sum2/2
  Sum2/1 -> Sum/2
  u/1 -> Integrator1/2, Gain/1  "u"
  Gain/1 -> Sum/1

== system Tmod_PID_ObsMej_Simulacion/Modulador de Torque/Ecuacion Tm 3.5, estrategia general ==
  Tm*' : Inport
  Id* : Inport  Port=2
  Constant : Constant  Value=lambda_m
  Divide : Product  Inputs=*/
  Gain : Gain  Gain=3/2 * Pp
  Gain1 : Gain  Gain=Ld-Lq
  Sum : Sum  Inputs=|++
  Iq*' : Outport
  wires:
  Tm*'/1 -> Divide/1
  Id*/1 -> Gain1/1
  Gain1/1 -> Sum/1
  Constant/1 -> Sum/2
  Sum/1 -> Gain/1
  Divide/1 -> Iq*'/1
  Gain/1 -> Divide/2

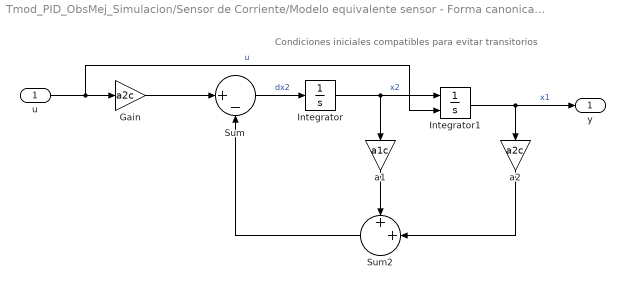
== system Tmod_PID_ObsMej_Simulacion/Sensor de Corriente/Modelo equivalente sensor - Forma canonica controlable ==
  note: Condiciones iniciales compatibles para evitar transitorios
  u : Inport
  Gain : Gain  Gain=a2c
  Integrator : Integrator
  Integrator1 : Integrator  InitialConditionSource=external
  Sum : Sum  Inputs=|+-
  Sum2 : Sum  Inputs=++|
  a1 : Gain  Gain=a1c
  a2 : Gain  Gain=a2c
  y : Outport
  wires:
  u/1 -> Integrator1/2, Gain/1  "u"
  Sum/1 -> Integrator/1  "dx2"
  Integrator/1 -> a1/1, Integrator1/1  "x2"
  a1/1 -> Sum2/1
  Integrator1/1 -> y/1, a2/1  "x1"
  a2/1 -> Sum2/2
  Sum2/1 -> Sum/2
  Gain/1 -> Sum/1

== system Tmod_PID_ObsMej_Simulacion/Sensor de Corriente/Modelo equivalente sensor - Forma canonica controlable1 ==
  note: Condiciones iniciales compatibles para evitar transitorios
  u : Inport
  Gain : Gain  Gain=a2c
  Integrator : Integrator
  Integrator1 : Integrator  InitialConditionSource=external
  Sum : Sum  Inputs=|+-
  Sum2 : Sum  Inputs=++|
  a1 : Gain  Gain=a1c
  a2 : Gain  Gain=a2c
  y : Outport
  wires:
  u/1 -> Integrator1/2, Gain/1  "u"
  Sum/1 -> Integrator/1  "dx2"
  Integrator/1 -> a1/1, Integrator1/1  "x2"
  a1/1 -> Sum2/1
  Integrator1/1 -> y/1, a2/1  "x1"
  a2/1 -> Sum2/2
  Sum2/1 -> Sum/2
  Gain/1 -> Sum/1

== system Tmod_PID_ObsMej_Simulacion/Sensor de Corriente/Modelo equivalente sensor - Forma canonica controlable2 ==
  note: Condiciones iniciales compatibles para evitar transitorios
  u : Inport
  Gain : Gain  Gain=a2c
  Integrator : Integrator
  Integrator1 : Integrator  InitialConditionSource=external
  Sum : Sum  Inputs=|+-
  Sum2 : Sum  Inputs=++|
  a1 : Gain  Gain=a1c
  a2 : Gain  Gain=a2c
  y : Outport
  wires:
  Sum/1 -> Integrator/1  "dx2"
  Integrator/1 -> a1/1, Integrator1/1  "x2"
  a1/1 -> Sum2/1
  Integrator1/1 -> y/1, a2/1  "x1"
  a2/1 -> Sum2/2
  Sum2/1 -> Sum/2
  u/1 -> Integrator1/2, Gain/1  "u"
  Gain/1 -> Sum/1

== system Tmod_PID_ObsMej_Simulacion/Sensor de posicion/Modelo equivalente sensor - Forma canonica controlable ==
  note: Condiciones iniciales compatibles para evitar transitorios
  u : Inport
  Gain : Gain  Gain=a2p
  Integrator : Integrator
  Integrator1 : Integrator  InitialConditionSource=external
  Sum : Sum  Inputs=|+-
  Sum2 : Sum  Inputs=++|
  a1 : Gain  Gain=a1p
  a2 : Gain  Gain=a2p
  y : Outport
  wires:
  u/1 -> Integrator1/2, Gain/1  "u"
  Sum/1 -> Integrator/1  "dx2"
  Integrator/1 -> a1/1, Integrator1/1  "x2"
  a1/1 -> Sum2/1
  Integrator1/1 -> y/1, a2/1  "x1"
  a2/1 -> Sum2/2
  Sum2/1 -> Sum/2
  Gain/1 -> Sum/1

== system Tmod_PID_ObsMej_Simulacion/sub_termico/Modelo equivalente sensor - Forma canonica controlable ==
  note: Condiciones iniciales compatibles para evitar transitorios
  u : Inport
  Integrator : Integrator  InitialConditionSource=external  InitialCondition=T_0
  Sum : Sum  Inputs=|+-
  a1 : Gain  Gain=a1t
  a1. : Gain  Gain=a1t
  y : Outport
  wires:
  u/1 -> a1./1  "u"
  Sum/1 -> Integrator/1  "dx1"
  Integrator/1 -> y/1, a1/1  "x1"
  a1/1 -> Sum/2
  a1./1 -> Sum/1

== matlab function Tmod_PID_ObsMej_Simulacion/inverse_park_transform ==
  data: fq input; fa output; fd input; f0 input; theta_r input; fb output; fc output
function [fa, fb, fc] =  inverse_park_transform(fq, fd, f0, theta_r)

ITP = [cos(theta_r)             sin(theta_r)           1;
       cos(theta_r - 2*pi/3)    sin(theta_r - 2*pi/3)  1;
       cos(theta_r + 2*pi/3)    sin(theta_r + 2*pi/3)  1];

abc = ITP*[fq; fd; f0];

fa = abc(1);
fb = abc(2);
fc = abc(3);
end

== matlab function Tmod_PID_ObsMej_Simulacion/inverse_park_transform1 ==
  data: fq input; fa output; fd input; f0 input; theta_r input; fb output; fc output
function [fa, fb, fc] =  inverse_park_transform(fq, fd, f0, theta_r)

ITP = [cos(theta_r)             sin(theta_r)           1;
       cos(theta_r - 2*pi/3)    sin(theta_r - 2*pi/3)  1;
       cos(theta_r + 2*pi/3)    sin(theta_r + 2*pi/3)  1];

abc = ITP*[fq; fd; f0];

fa = abc(1);
fb = abc(2);
fc = abc(3);
end

== matlab function Tmod_PID_ObsMej_Simulacion/park_transform ==
  data: fa input; fq output; fb input; fc input; theta_r input; fd output; f0 output
function [fq, fd, f0] =  park_transform(fa, fb, fc, theta_r)
    
TP = 2/3*[cos(theta_r)  cos(theta_r - 2*pi/3)   cos(theta_r + 2*pi/3);
          sin(theta_r)  sin(theta_r - 2*pi/3)   sin(theta_r + 2*pi/3);
          1/2           1/2                     1/2];
     
qd0 = TP*[fa; fb; fc];

fq = qd0(1);
fd = qd0(2);
f0 = qd0(3);
end

== matlab function Tmod_PID_ObsMej_Simulacion/park_transform1 ==
  data: fa input; fq output; fb input; fc input; theta_r input; fd output; f0 output
function [fq, fd, f0] =  park_transform(fa, fb, fc, theta_r)
    
TP = 2/3*[cos(theta_r)  cos(theta_r - 2*pi/3)   cos(theta_r + 2*pi/3);
          sin(theta_r)  sin(theta_r - 2*pi/3)   sin(theta_r + 2*pi/3);
          1/2           1/2                     1/2];
     
qd0 = TP*[fa; fb; fc];

fq = qd0(1);
fd = qd0(2);
f0 = qd0(3);
end
